simulink model "Final_ECM_App"  (R2021b)
settings: Solver=FixedStepAuto  StartTime=0.0  StopTime=max(Time)  FixedStep=0.009  RelTol=1e-3  AbsTol=1e-3
undefined symbols (not defined in the file or in its folder): C1, DiscIntNeverNeededParam, Nominal_Capacity, R0, R0_SOC_para, R1, R1_SOC_para, VOC, VOC_SOC_para
libraries: nesl_utility x10, fl_lib x9, ee_lib x1
settings Model: Creator=amin najafi  LastModifiedBy=amin najafi
settings SolverCC: AutoScaleAbsTol=off  AlgebraicLoopSolver=TrustRegion
settings DebuggingCC: SymbolicDimsDataTypeCodeGenerationDiagnostic=none  SFMachineParentedDataDiag=warning
settings SFSimCC: CustomCodeUndefinedFunction=UseInterfaceOnly
settings SimscapeCC: SimscapeLogType=all  SimscapeLogSimulationStatistics=on  SimscapeLogDataHistory=10000

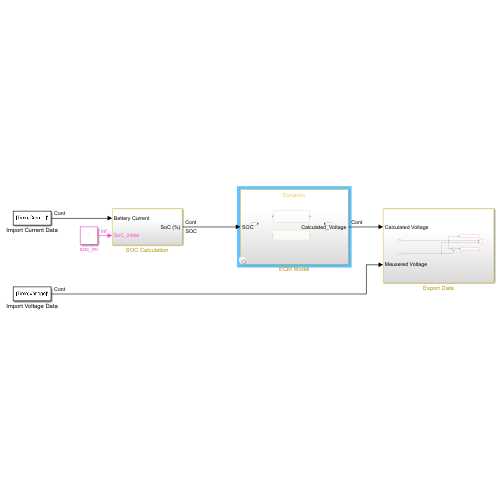
[thumbnail: Simulink's stored preview of the top-level diagram]
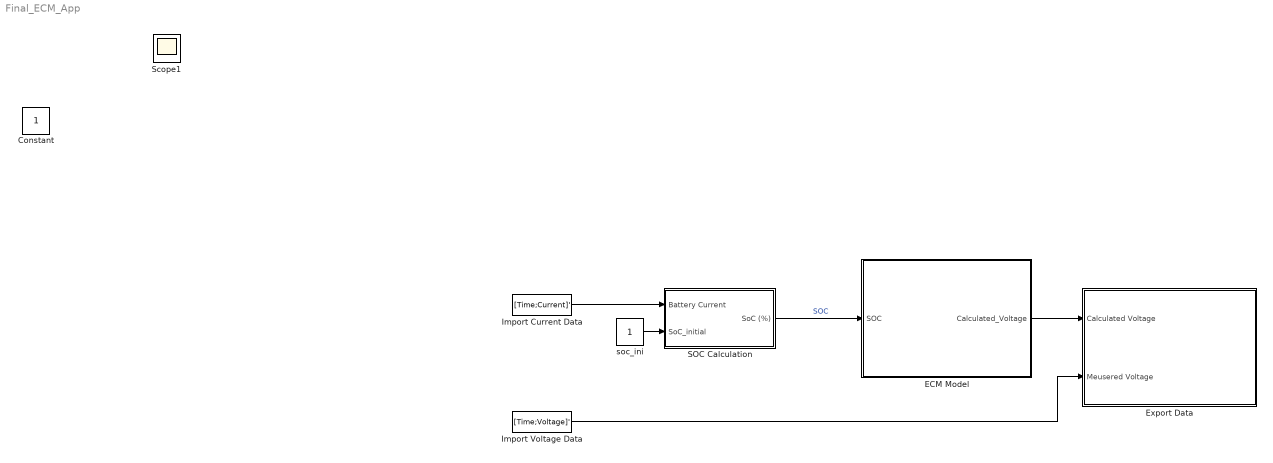
== system Final_ECM_App ==
  ECM Model : Subsystem  Variant=on
  Export Data : Subsystem
  Import Current Data : FromWorkspace  VariableName=[Time;Current]'  OutDataTypeStr=double  SampleTime=-1
  Import Voltage Data : FromWorkspace  VariableName=[Time;Voltage]'  OutDataTypeStr=double  SampleTime=-1
  SOC Calculation : Subsystem
  soc_ini : Constant
  Constant : Constant  IOType=siggen
  Scope1 : Scope
  wires:
  soc_ini/1 -> SOC Calculation/2(SoC_initial)
  SOC Calculation/1(SoC (%)) -> ECM Model/1(SOC)  "SOC"
  Import Current Data/1 -> SOC Calculation/1(Battery Current)
  ECM Model/1(Calculated_Voltage) -> Export Data/1(Calculated Voltage)
  Import Voltage Data/1 -> Export Data/2(Meusered Voltage)

== system Final_ECM_App/ECM Model ==
  SOC : Inport
  Dynamic : Subsystem  VariantControl=Architecture ==1
  Static : Subsystem  VariantControl=Architecture == 0
  Calculated_Voltage : Outport

== system Final_ECM_App/Export Data ==
  Calculated Voltage : Inport
  Meusered Voltage : Inport  Port=2
  Export Error Voltage Data : ToWorkspace  VariableName=Error_Voltage  SaveFormat=Timeseries  SampleTime=-1
      settings: Save2DSignal=2-D array (concatenate along first dimension)
  Export Voltage Data : ToWorkspace  VariableName=Calculated_Voltage  SaveFormat=Timeseries  SampleTime=-1
      settings: Save2DSignal=2-D array (concatenate along first dimension)
  Scope1 : Scope  NumInputPorts=2
  Sum : Sum  Inputs=|+-
  wires:
  Calculated Voltage/1 -> Scope1/1, Export Voltage Data/1, Sum/1
  Sum/1 -> Export Error Voltage Data/1
  Meusered Voltage/1 -> Scope1/2, Sum/2

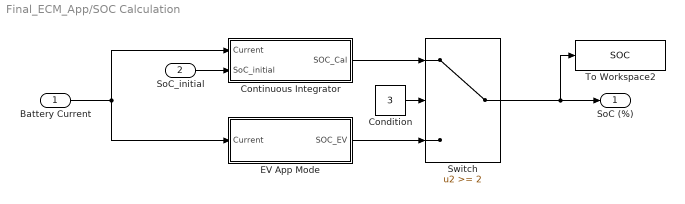
== system Final_ECM_App/SOC Calculation ==
  Battery Current : Inport
  SoC_initial : Inport  Port=2
  Condition : Constant  Value=3
  "Continuous Integrator " : Subsystem
  EV App Mode : Subsystem
  Switch : Switch  Threshold=2
  To Workspace2 : ToWorkspace  VariableName=SOC  SaveFormat=Timeseries  SampleTime=-1
      settings: Save2DSignal=2-D array (concatenate along first dimension)
  SoC (%) : Outport
  wires:
  Battery Current/1 -> EV App Mode/1(Current), "Continuous Integrator "/1(Current)
  SoC_initial/1 -> "Continuous Integrator "/2(SoC_initial)
  "Continuous Integrator "/1(SOC_Cal) -> Switch/1
  EV App Mode/1(SOC_EV) -> Switch/3
  Switch/1 -> SoC (%)/1, To Workspace2/1
  Condition/1 -> Switch/2

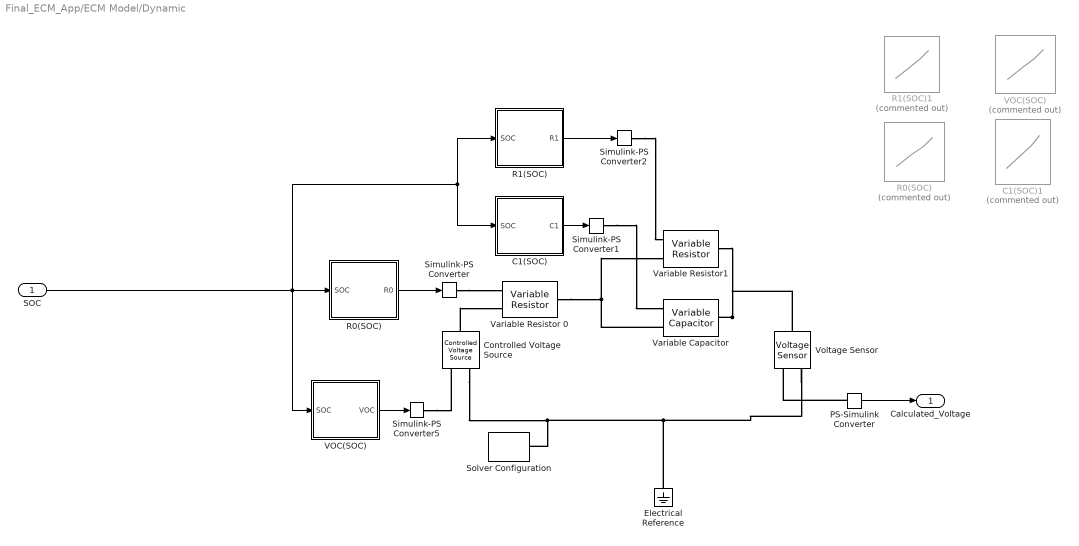
== system Final_ECM_App/ECM Model/Dynamic ==
  SOC : Inport
  "C1(SOC) " : Subsystem
  C1(SOC)1 : Lookup_n-D  Commented=on  NumberOfTableDimensions=1  BreakpointsForDimension1=[0 10 20 30 40 50 60 70 80 90 100]  Table=[C1]  InternalRulePriority=Speed  RndMeth=Simplest  InputSameDT=on
  Controlled Voltage Source : fl_lib/Electrical/Electrical Sources/Controlled Voltage Source
  Electrical Reference : fl_lib/Electrical/Electrical Elements/Electrical Reference
  PS-Simulink Converter : nesl_utility/PS-Simulink Converter  PhysicalDomain=network_engine_domain  SubClassName=ps_output  LeftPortType=input  RightPortType=output  PseudoPeriodic=off  Frequencies=[]  Unit=inherit  AffineConversion=off
      settings: SourceProductBaseCode=PW,SS
  R0(SOC) : Lookup_n-D  Commented=on  NumberOfTableDimensions=1  BreakpointsForDimension1=[0 10 20 30 40 50 60 70 80 90 100]  Table=[R0]  InternalRulePriority=Speed  RndMeth=Simplest  InputSameDT=on
  "R0(SOC)  " : Subsystem
  "R1(SOC)   " : Subsystem
  R1(SOC)1 : Lookup_n-D  Commented=on  NumberOfTableDimensions=1  BreakpointsForDimension1=[0 10 20 30 40 50 60 70 80 90 100]  Table=[R1]  InternalRulePriority=Speed  RndMeth=Simplest  InputSameDT=on
  Simulink-PS Converter{,1..2,5} (4 alike) : nesl_utility/Simulink-PS Converter  PhysicalDomain=network_engine_domain  SubClassName=ps_input  LeftPortType=input  RightPortType=output  PseudoPeriodic=off  Frequencies=[]  NoiseDistribution=none  NoiseParameters=[]  Unit=1  AffineConversion=off  FilteringAndDerivatives=provide  SimscapeFilterOrder=1  InputFilterTimeConstant=0.001  UdotUserProvided=0
      settings: SourceProductBaseCode=PW,SS
  Solver Configuration : nesl_utility/Solver Configuration  PhysicalDomain=network_engine_domain  SubClassName=solver  LeftPortType=input  RightPortType=generic  Tones=[]  Harmonics=[]  SimulateNoise=off  Profile=off  UseLocalSampling=off  EnableSwitchedLinearOptims=on  FrequencyDomain=off  UseCCode=off  RelTol=0.001  AbsTol=1e-06  MinStep=1e-09  ToWorkspace=off  RevertToSquareIcSolve=off  NumHomotopyIterations=100  PhasorMode=off  PhasorModeNumHarmonics=1  DoDC=off  ResidualTolerance=1e-09  UseLocalSolver=off  LocalSolverChoice=NE_BACKWARD_EULER_ADVANCER  LocalSolverSampleTime=0.001  DoFixedCost=off  MaxNonlinIter=3  MaxModeIter=2  ComputeImpulses=off  ImpulseIterations=2  LinearAlgebra=auto  EquationFormulation=NE_TIME_EF  DelaysMemoryBudget=1024  AutomaticFiltering=on  FilteringTimeConstant=0.001  PartitionStorageMethod=AS_NEEDED  PartitionMemoryBudget=1024  PartitionMethod=ROBUST
      settings: SourceProductBaseCode=PW,SS
  VOC(SOC) : Lookup_n-D  Commented=on  NumberOfTableDimensions=1  BreakpointsForDimension1=[0 10 20 30 40 50 60 70 80 90 100]  Table=[VOC]  InternalRulePriority=Speed  RndMeth=Simplest  InputSameDT=on
  "VOC(SOC) " : Subsystem
  Variable Capacitor : ee_lib/Passive/Variable Capacitor  prm=2  Cmin=1e-9 F  r=1e-6 Ohm  v0=0 V  q0=0 C
      settings: SourceProductBaseCode=PS  InternalSimscapePortConfiguration="{\"Bottom\":[],\"Left\":[{\"id\":\"C\",\"label\":\"C\",\"type\":\"input\"},{\"id\":\"p\",\"label\":\"+\",\"type\":\"foundation.electrical.electrical\"}],\"Right\":[{\"id\":\"n\",\"label\":\"-\",\"type\":\"foundation.electrical.electrical\"}],\"Top\":[]}"
  Variable Resistor 0 : fl_lib/Electrical/Electrical Elements/Variable Resistor  Rmin=0 Ohm  i_specify=off  i_priority=None  i=0 A  i_nominal_specify=off  i_nominal_unit=A  i_nominal_value=1  v_specify=off  v_priority=None  v=0 V  v_nominal_specify=off  v_nominal_unit=V  v_nominal_value=1
  Variable Resistor1 : fl_lib/Electrical/Electrical Elements/Variable Resistor  Rmin=0 Ohm  i_specify=off  i_priority=None  i=0 A  i_nominal_specify=off  i_nominal_unit=A  i_nominal_value=1  v_specify=off  v_priority=None  v=0 V  v_nominal_specify=off  v_nominal_unit=V  v_nominal_value=1
  Voltage Sensor : fl_lib/Electrical/Electrical Sensors/Voltage Sensor
  Calculated_Voltage : Outport
  wires:
  PS-Simulink Converter/1 -> Calculated_Voltage/1
  SOC/1 -> "C1(SOC) "/1(SOC), "R1(SOC)   "/1(SOC), "R0(SOC)  "/1(SOC), "VOC(SOC) "/1(SOC)
  "C1(SOC) "/1(C1) -> Simulink-PS Converter1/1
  "R1(SOC)   "/1(R1) -> Simulink-PS Converter2/1
  "R0(SOC)  "/1(R0) -> Simulink-PS Converter/1
  "VOC(SOC) "/1(VOC) -> Simulink-PS Converter5/1
  connections:
  Variable Capacitor/RConn1 -- Voltage Sensor/LConn1 -- Variable Resistor1/RConn1
  Variable Capacitor/LConn2 -- Variable Resistor 0/RConn1 -- Variable Resistor1/LConn2
  Simulink-PS Converter/RConn1 -- Variable Resistor 0/LConn1
  Simulink-PS Converter5/RConn1 -- Controlled Voltage Source/RConn1
  Simulink-PS Converter1/RConn1 -- Variable Capacitor/LConn1
  Controlled Voltage Source/LConn1 -- Variable Resistor 0/LConn2
  Simulink-PS Converter2/RConn1 -- Variable Resistor1/LConn1
  PS-Simulink Converter/LConn1 -- Voltage Sensor/RConn1
  Voltage Sensor/RConn2 -- Controlled Voltage Source/RConn2 -- Solver Configuration/RConn1 -- Electrical Reference/LConn1

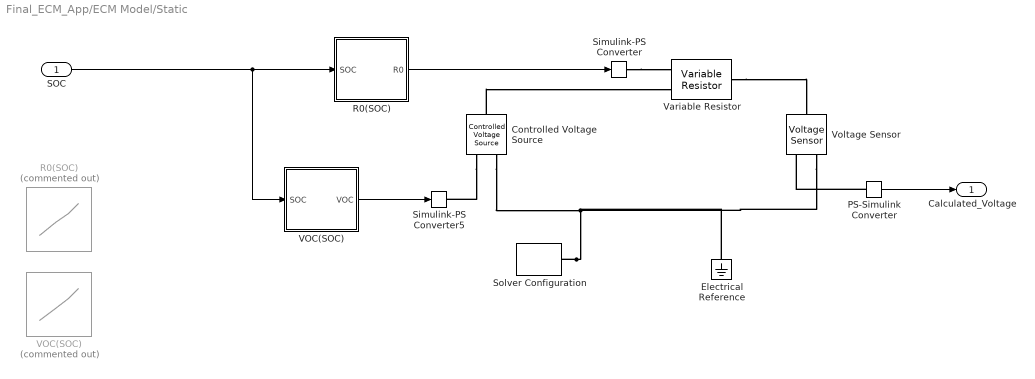
== system Final_ECM_App/ECM Model/Static ==
  SOC : Inport
  Controlled Voltage Source : fl_lib/Electrical/Electrical Sources/Controlled Voltage Source
  Electrical Reference : fl_lib/Electrical/Electrical Elements/Electrical Reference
  PS-Simulink Converter : nesl_utility/PS-Simulink Converter  PhysicalDomain=network_engine_domain  SubClassName=ps_output  LeftPortType=input  RightPortType=output  PseudoPeriodic=off  Frequencies=[]  Unit=inherit  AffineConversion=off
      settings: SourceProductBaseCode=PW,SS
  R0(SOC) : Lookup_n-D  Commented=on  NumberOfTableDimensions=1  BreakpointsForDimension1=[0 10 20 30 40 50 60 70 80 90 100]  Table=[R0]  InternalRulePriority=Speed  RndMeth=Simplest  InputSameDT=on
  "R0(SOC) " : Subsystem
  Simulink-PS Converter : nesl_utility/Simulink-PS Converter  PhysicalDomain=network_engine_domain  SubClassName=ps_input  LeftPortType=input  RightPortType=output  PseudoPeriodic=off  Frequencies=[]  NoiseDistribution=none  NoiseParameters=[]  Unit=1  AffineConversion=off  FilteringAndDerivatives=provide  SimscapeFilterOrder=1  InputFilterTimeConstant=0.001  UdotUserProvided=0
      settings: SourceProductBaseCode=PW,SS
  Simulink-PS Converter5 : nesl_utility/Simulink-PS Converter  PhysicalDomain=network_engine_domain  SubClassName=ps_input  LeftPortType=input  RightPortType=output  PseudoPeriodic=off  Frequencies=[]  NoiseDistribution=none  NoiseParameters=[]  Unit=1  AffineConversion=off  FilteringAndDerivatives=provide  SimscapeFilterOrder=1  InputFilterTimeConstant=0.001  UdotUserProvided=0
      settings: SourceProductBaseCode=PW,SS
  Solver Configuration : nesl_utility/Solver Configuration  PhysicalDomain=network_engine_domain  SubClassName=solver  LeftPortType=input  RightPortType=generic  Tones=[]  Harmonics=[]  SimulateNoise=off  Profile=off  UseLocalSampling=off  EnableSwitchedLinearOptims=on  FrequencyDomain=off  UseCCode=off  RelTol=0.001  AbsTol=1e-06  MinStep=1e-09  ToWorkspace=off  RevertToSquareIcSolve=off  NumHomotopyIterations=100  PhasorMode=off  PhasorModeNumHarmonics=1  DoDC=off  ResidualTolerance=1e-09  UseLocalSolver=off  LocalSolverChoice=NE_BACKWARD_EULER_ADVANCER  LocalSolverSampleTime=0.001  DoFixedCost=off  MaxNonlinIter=3  MaxModeIter=2  ComputeImpulses=off  ImpulseIterations=2  LinearAlgebra=auto  EquationFormulation=NE_TIME_EF  DelaysMemoryBudget=1024  AutomaticFiltering=on  FilteringTimeConstant=0.001  PartitionStorageMethod=AS_NEEDED  PartitionMemoryBudget=1024  PartitionMethod=ROBUST
      settings: SourceProductBaseCode=PW,SS
  VOC(SOC) : Lookup_n-D  Commented=on  NumberOfTableDimensions=1  BreakpointsForDimension1=[0 10 20 30 40 50 60 70 80 90 100]  Table=[VOC]  InternalRulePriority=Speed  RndMeth=Simplest  InputSameDT=on
  "VOC(SOC) " : Subsystem
  Variable Resistor : fl_lib/Electrical/Electrical Elements/Variable Resistor  Rmin=0 Ohm  i_specify=off  i_priority=None  i=0 A  i_nominal_specify=off  i_nominal_unit=A  i_nominal_value=1  v_specify=off  v_priority=None  v=0 V  v_nominal_specify=off  v_nominal_unit=V  v_nominal_value=1
  Voltage Sensor : fl_lib/Electrical/Electrical Sensors/Voltage Sensor
  Calculated_Voltage : Outport
  wires:
  PS-Simulink Converter/1 -> Calculated_Voltage/1
  SOC/1 -> "R0(SOC) "/1(SOC), "VOC(SOC) "/1(SOC)
  "VOC(SOC) "/1(VOC) -> Simulink-PS Converter5/1
  "R0(SOC) "/1(R0) -> Simulink-PS Converter/1
  connections:
  Solver Configuration/RConn1 -- Controlled Voltage Source/RConn2 -- Voltage Sensor/RConn2 -- Electrical Reference/LConn1
  Controlled Voltage Source/LConn1 -- Variable Resistor/LConn2
  PS-Simulink Converter/LConn1 -- Voltage Sensor/RConn1
  Simulink-PS Converter/RConn1 -- Variable Resistor/LConn1
  Controlled Voltage Source/RConn1 -- Simulink-PS Converter5/RConn1
  Variable Resistor/RConn1 -- Voltage Sensor/LConn1

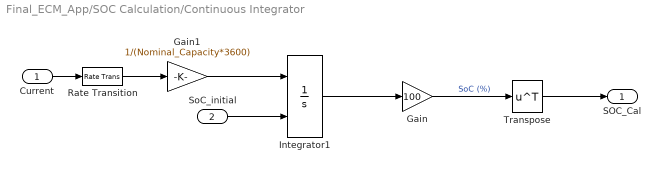
== system Final_ECM_App/SOC Calculation/Continuous Integrator  ==
  Current : Inport
  SoC_initial : Inport  Port=2
  Gain : Gain  Gain=100
  Gain1 : Gain  Gain=1/(Nominal_Capacity*3600)
  Integrator1 : Integrator  InitialConditionSource=external  LimitOutput=on  UpperSaturationLimit=1  LowerSaturationLimit=0  IgnoreLimit=on
  Rate Transition : RateTransition  Deterministic=off
  Transpose : Math  Operator=transpose  SaturateOnIntegerOverflow=on
  SOC_Cal : Outport
  wires:
  SoC_initial/1 -> Integrator1/2
  Rate Transition/1 -> Gain1/1
  Integrator1/1 -> Gain/1
  Gain/1 -> Transpose/1  "SoC (%)"
  Current/1 -> Rate Transition/1
  Gain1/1 -> Integrator1/1
  Transpose/1 -> SOC_Cal/1

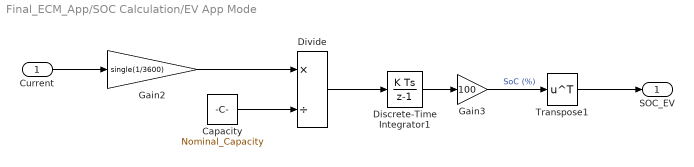
== system Final_ECM_App/SOC Calculation/EV App Mode ==
  Current : Inport
  Capacity : Constant  Value=Nominal_Capacity
  Discrete-Time Integrator1 : DiscreteIntegrator  InitialCondition=single(1)  SampleTime=-1  LimitOutput=on  UpperSaturationLimit=1  LowerSaturationLimit=0  ICPrevOutput=DiscIntNeverNeededParam  ICPrevScaledInput=DiscIntNeverNeededParam
  Divide : Product  Inputs=*/
  Gain2 : Gain  Gain=single(1/3600)
  Gain3 : Gain  Gain=100
  Transpose1 : Math  Operator=transpose  SaturateOnIntegerOverflow=on
  SOC_EV : Outport
  wires:
  Capacity/1 -> Divide/2
  Discrete-Time Integrator1/1 -> Gain3/1
  Transpose1/1 -> SOC_EV/1
  Divide/1 -> Discrete-Time Integrator1/1
  Gain2/1 -> Divide/1
  Current/1 -> Gain2/1
  Gain3/1 -> Transpose1/1  "SoC (%)"

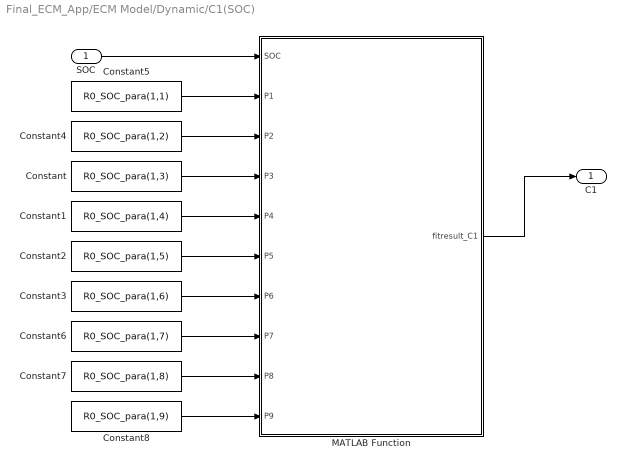
== system Final_ECM_App/ECM Model/Dynamic/C1(SOC)  ==
  SOC : Inport
  Constant : Constant  Value=R0_SOC_para(1,3)
  Constant1 : Constant  Value=R0_SOC_para(1,4)
  Constant2 : Constant  Value=R0_SOC_para(1,5)
  Constant3 : Constant  Value=R0_SOC_para(1,6)
  Constant4 : Constant  Value=R0_SOC_para(1,2)
  Constant5 : Constant  Value=R0_SOC_para(1,1)
  Constant6 : Constant  Value=R0_SOC_para(1,7)
  Constant7 : Constant  Value=R0_SOC_para(1,8)
  Constant8 : Constant  Value=R0_SOC_para(1,9)
  MATLAB Function : MATLAB Function  TreatAsAtomicUnit=on
  C1 : Outport
  wires:
  MATLAB Function/1(fitresult_C1) -> C1/1
  SOC/1 -> MATLAB Function/1(SOC)
  Constant5/1 -> MATLAB Function/2(P1)
  Constant4/1 -> MATLAB Function/3(P2)
  Constant/1 -> MATLAB Function/4(P3)
  Constant1/1 -> MATLAB Function/5(P4)
  Constant2/1 -> MATLAB Function/6(P5)
  Constant3/1 -> MATLAB Function/7(P6)
  Constant6/1 -> MATLAB Function/8(P7)
  Constant7/1 -> MATLAB Function/9(P8)
  Constant8/1 -> MATLAB Function/10(P9)

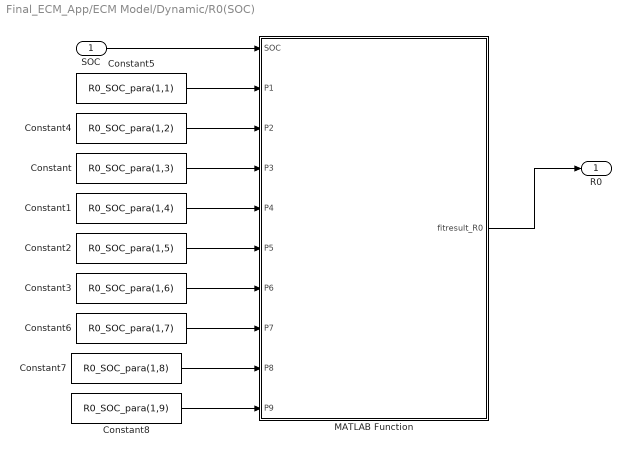
== system Final_ECM_App/ECM Model/Dynamic/R0(SOC)   ==
  SOC : Inport
  Constant : Constant  Value=R0_SOC_para(1,3)
  Constant1 : Constant  Value=R0_SOC_para(1,4)
  Constant2 : Constant  Value=R0_SOC_para(1,5)
  Constant3 : Constant  Value=R0_SOC_para(1,6)
  Constant4 : Constant  Value=R0_SOC_para(1,2)
  Constant5 : Constant  Value=R0_SOC_para(1,1)
  Constant6 : Constant  Value=R0_SOC_para(1,7)
  Constant7 : Constant  Value=R0_SOC_para(1,8)
  Constant8 : Constant  Value=R0_SOC_para(1,9)
  MATLAB Function : MATLAB Function  TreatAsAtomicUnit=on
  R0 : Outport
  wires:
  MATLAB Function/1(fitresult_R0) -> R0/1
  SOC/1 -> MATLAB Function/1(SOC)
  Constant5/1 -> MATLAB Function/2(P1)
  Constant4/1 -> MATLAB Function/3(P2)
  Constant/1 -> MATLAB Function/4(P3)
  Constant1/1 -> MATLAB Function/5(P4)
  Constant2/1 -> MATLAB Function/6(P5)
  Constant3/1 -> MATLAB Function/7(P6)
  Constant8/1 -> MATLAB Function/10(P9)
  Constant7/1 -> MATLAB Function/9(P8)
  Constant6/1 -> MATLAB Function/8(P7)

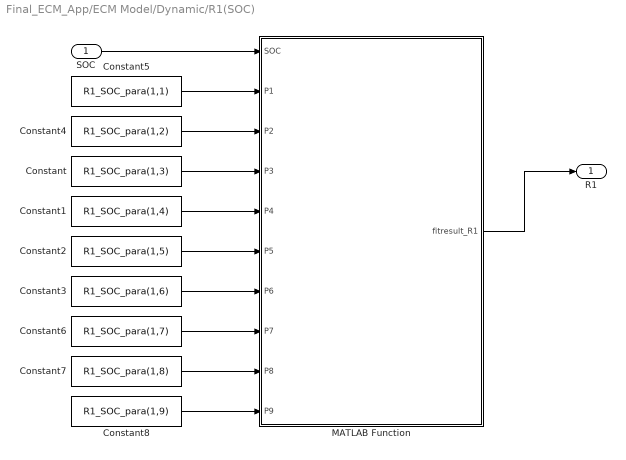
== system Final_ECM_App/ECM Model/Dynamic/R1(SOC)    ==
  SOC : Inport
  Constant : Constant  Value=R1_SOC_para(1,3)
  Constant1 : Constant  Value=R1_SOC_para(1,4)
  Constant2 : Constant  Value=R1_SOC_para(1,5)
  Constant3 : Constant  Value=R1_SOC_para(1,6)
  Constant4 : Constant  Value=R1_SOC_para(1,2)
  Constant5 : Constant  Value=R1_SOC_para(1,1)
  Constant6 : Constant  Value=R1_SOC_para(1,7)
  Constant7 : Constant  Value=R1_SOC_para(1,8)
  Constant8 : Constant  Value=R1_SOC_para(1,9)
  MATLAB Function : MATLAB Function  TreatAsAtomicUnit=on
  R1 : Outport
  wires:
  Constant3/1 -> MATLAB Function/7(P6)
  Constant2/1 -> MATLAB Function/6(P5)
  Constant1/1 -> MATLAB Function/5(P4)
  Constant/1 -> MATLAB Function/4(P3)
  Constant4/1 -> MATLAB Function/3(P2)
  Constant5/1 -> MATLAB Function/2(P1)
  SOC/1 -> MATLAB Function/1(SOC)
  MATLAB Function/1(fitresult_R1) -> R1/1
  Constant6/1 -> MATLAB Function/8(P7)
  Constant7/1 -> MATLAB Function/9(P8)
  Constant8/1 -> MATLAB Function/10(P9)

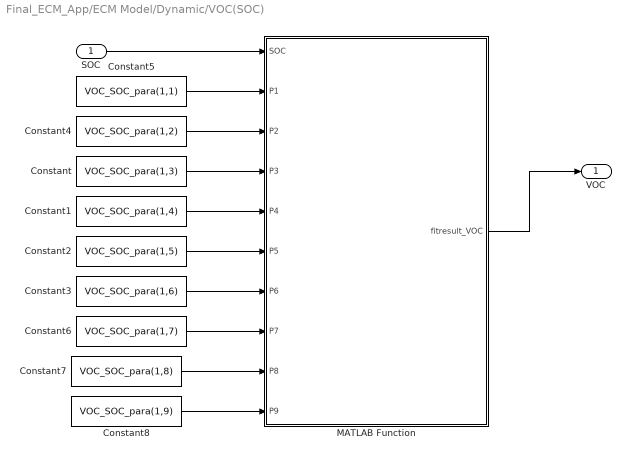
== system Final_ECM_App/ECM Model/Dynamic/VOC(SOC)  ==
  SOC : Inport
  Constant : Constant  Value=VOC_SOC_para(1,3)
  Constant1 : Constant  Value=VOC_SOC_para(1,4)
  Constant2 : Constant  Value=VOC_SOC_para(1,5)
  Constant3 : Constant  Value=VOC_SOC_para(1,6)
  Constant4 : Constant  Value=VOC_SOC_para(1,2)
  Constant5 : Constant  Value=VOC_SOC_para(1,1)
  Constant6 : Constant  Value=VOC_SOC_para(1,7)
  Constant7 : Constant  Value=VOC_SOC_para(1,8)
  Constant8 : Constant  Value=VOC_SOC_para(1,9)
  MATLAB Function : MATLAB Function  TreatAsAtomicUnit=on
  VOC : Outport
  wires:
  Constant3/1 -> MATLAB Function/7(P6)
  Constant2/1 -> MATLAB Function/6(P5)
  Constant1/1 -> MATLAB Function/5(P4)
  Constant/1 -> MATLAB Function/4(P3)
  Constant4/1 -> MATLAB Function/3(P2)
  Constant5/1 -> MATLAB Function/2(P1)
  SOC/1 -> MATLAB Function/1(SOC)
  MATLAB Function/1(fitresult_VOC) -> VOC/1
  Constant6/1 -> MATLAB Function/8(P7)
  Constant7/1 -> MATLAB Function/9(P8)
  Constant8/1 -> MATLAB Function/10(P9)

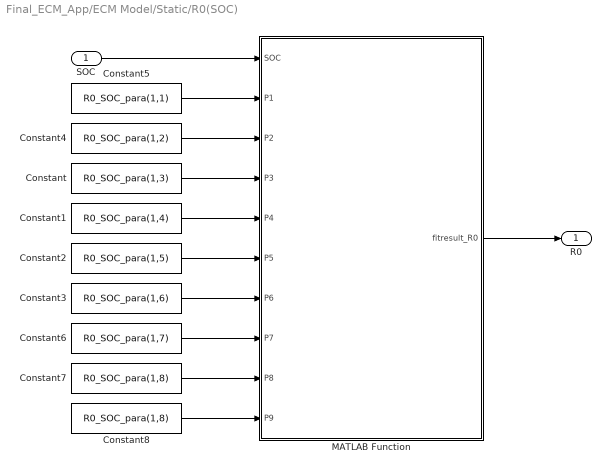
== system Final_ECM_App/ECM Model/Static/R0(SOC)  ==
  SOC : Inport
  Constant : Constant  Value=R0_SOC_para(1,3)
  Constant1 : Constant  Value=R0_SOC_para(1,4)
  Constant2 : Constant  Value=R0_SOC_para(1,5)
  Constant3 : Constant  Value=R0_SOC_para(1,6)
  Constant4 : Constant  Value=R0_SOC_para(1,2)
  Constant5 : Constant  Value=R0_SOC_para(1,1)
  Constant6 : Constant  Value=R0_SOC_para(1,7)
  Constant7 : Constant  Value=R0_SOC_para(1,8)
  Constant8 : Constant  Value=R0_SOC_para(1,8)
  MATLAB Function : MATLAB Function  TreatAsAtomicUnit=on
  R0 : Outport
  wires:
  Constant3/1 -> MATLAB Function/7(P6)
  Constant2/1 -> MATLAB Function/6(P5)
  Constant1/1 -> MATLAB Function/5(P4)
  Constant/1 -> MATLAB Function/4(P3)
  Constant4/1 -> MATLAB Function/3(P2)
  Constant5/1 -> MATLAB Function/2(P1)
  SOC/1 -> MATLAB Function/1(SOC)
  MATLAB Function/1(fitresult_R0) -> R0/1
  Constant6/1 -> MATLAB Function/8(P7)
  Constant7/1 -> MATLAB Function/9(P8)
  Constant8/1 -> MATLAB Function/10(P9)

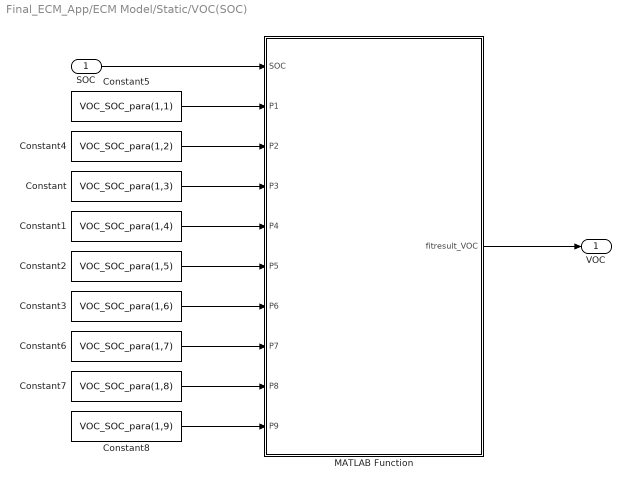
== system Final_ECM_App/ECM Model/Static/VOC(SOC)  ==
  SOC : Inport
  Constant : Constant  Value=VOC_SOC_para(1,3)
  Constant1 : Constant  Value=VOC_SOC_para(1,4)
  Constant2 : Constant  Value=VOC_SOC_para(1,5)
  Constant3 : Constant  Value=VOC_SOC_para(1,6)
  Constant4 : Constant  Value=VOC_SOC_para(1,2)
  Constant5 : Constant  Value=VOC_SOC_para(1,1)
  Constant6 : Constant  Value=VOC_SOC_para(1,7)
  Constant7 : Constant  Value=VOC_SOC_para(1,8)
  Constant8 : Constant  Value=VOC_SOC_para(1,9)
  MATLAB Function : MATLAB Function  TreatAsAtomicUnit=on
  VOC : Outport
  wires:
  MATLAB Function/1(fitresult_VOC) -> VOC/1
  SOC/1 -> MATLAB Function/1(SOC)
  Constant5/1 -> MATLAB Function/2(P1)
  Constant4/1 -> MATLAB Function/3(P2)
  Constant/1 -> MATLAB Function/4(P3)
  Constant1/1 -> MATLAB Function/5(P4)
  Constant2/1 -> MATLAB Function/6(P5)
  Constant3/1 -> MATLAB Function/7(P6)
  Constant6/1 -> MATLAB Function/8(P7)
  Constant7/1 -> MATLAB Function/9(P8)
  Constant8/1 -> MATLAB Function/10(P9)

== matlab function Final_ECM_App/ECM Model/Static/R0(SOC) /MATLAB Function ==
  data: SOC input; fitresult_R0 output; P1 input; P2 input; P3 input; P4 input; P5 input; P6 input; P7 input; P8 input; P9 input
function fitresult_R0  = func(SOC,P1,P2,P3,P4,P5,P6,P7,P8,P9)
fitresult_R0 = P1*SOC^8 + P2*SOC^7 + P3*SOC^6 + P4*SOC^5 + P5*SOC^4 + P6*SOC^3+ P7*SOC^2+ P8*SOC+ P9;
end

== matlab function Final_ECM_App/ECM Model/Static/VOC(SOC) /MATLAB Function ==
  data: SOC input; fitresult_VOC output; P1 input; P2 input; P3 input; P4 input; P5 input; P6 input; P7 input; P8 input; P9 input
function fitresult_VOC  = func(SOC,P1,P2,P3,P4,P5,P6,P7,P8,P9)
    fitresult_VOC = P1*SOC^8 + P2*SOC^7 + P3*SOC^6 + P4*SOC^5 + P5*SOC^4 + P6*SOC^3+ P7*SOC^2+ P8*SOC+ P9;
end

== matlab function Final_ECM_App/ECM Model/Dynamic/R0(SOC)  /MATLAB Function ==
  data: SOC input; fitresult_R0 output; P1 input; P2 input; P3 input; P4 input; P5 input; P6 input; P7 input; P8 input; P9 input
function fitresult_R0  = func(SOC,P1,P2,P3,P4,P5,P6,P7,P8,P9)
fitresult_R0 = P1*SOC^8 + P2*SOC^7 + P3*SOC^6 + P4*SOC^5 + P5*SOC^4 + P6*SOC^3+ P7*SOC^2+ P8*SOC+ P9;
end

== matlab function Final_ECM_App/ECM Model/Dynamic/VOC(SOC) /MATLAB Function ==
  data: SOC input; fitresult_VOC output; P1 input; P2 input; P3 input; P4 input; P5 input; P6 input; P7 input; P8 input; P9 input
function fitresult_VOC  = func(SOC,P1,P2,P3,P4,P5,P6,P7,P8,P9)
    fitresult_VOC = P1*SOC^8 + P2*SOC^7 + P3*SOC^6 + P4*SOC^5 + P5*SOC^4 + P6*SOC^3+ P7*SOC^2+ P8*SOC+ P9;
end

== matlab function Final_ECM_App/ECM Model/Dynamic/R1(SOC)   /MATLAB Function ==
  data: SOC input; fitresult_R1 output; P1 input; P2 input; P3 input; P4 input; P5 input; P6 input; P7 input; P8 input; P9 input
function fitresult_R1  = func(SOC,P1,P2,P3,P4,P5,P6,P7,P8,P9)
fitresult_R1 = P1*SOC^8 + P2*SOC^7 + P3*SOC^6 + P4*SOC^5 + P5*SOC^4 + P6*SOC^3+ P7*SOC^2+ P8*SOC+ P9;
end

== matlab function Final_ECM_App/ECM Model/Dynamic/C1(SOC) /MATLAB Function ==
  data: SOC input; fitresult_C1 output; P1 input; P2 input; P3 input; P4 input; P5 input; P6 input; P7 input; P8 input; P9 input
function fitresult_C1  = func(SOC,P1,P2,P3,P4,P5,P6,P7,P8,P9)
fitresult_C1 = P1*SOC^8 + P2*SOC^7 + P3*SOC^6 + P4*SOC^5 + P5*SOC^4 + P6*SOC^3+ P7*SOC^2+ P8*SOC+ P9;
end
